simulink model "Ideal_Push_pull"  (R2022b)
settings: Solver=VariableStepAuto  StartTime=0.0  StopTime=0.1  FixedStep=1/2e6  RelTol=1e-3
libraries: spsSeriesRLCBranchLib x4, spsVoltageMeasurementLib x3, spsCurrentMeasurementLib x2, spsDiodeLib x2, spsIdealSwitchLib x2, spsDCVoltageSourceLib x1, spsGroundLib x1, spsMultiWindingTransformerLib x1, spspowerguiLib x1
settings Model: Creator=smlmc  LastModifiedBy=smlmc
settings DebuggingCC: MaskedZcDiagnostic=none  IgnoredZcDiagnostic=none

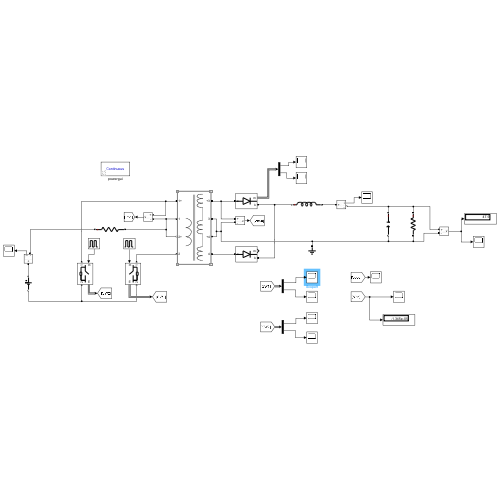
[thumbnail: Simulink's stored preview of the top-level diagram]
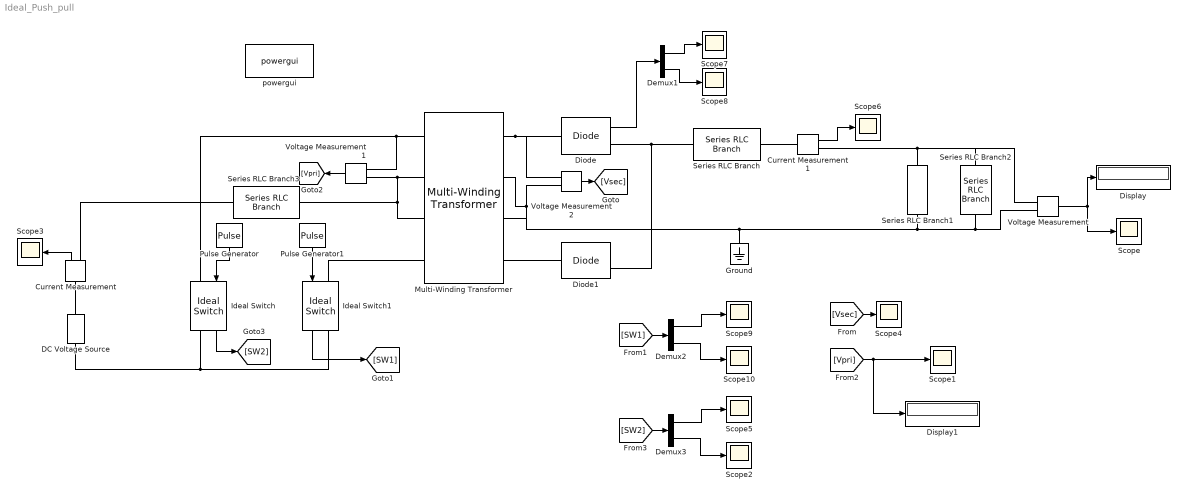
== system Ideal_Push_pull ==
  Current Measurement : spsCurrentMeasurementLib/Current Measurement  PhasorSimulation=off  OutputType=Complex  PSBequivalent=0
  Current Measurement1 : spsCurrentMeasurementLib/Current Measurement  PhasorSimulation=off  OutputType=Complex  PSBequivalent=0
  DC Voltage Source : spsDCVoltageSourceLib/DC Voltage Source  Amplitude=12  Measurements=None
  Demux1 : Demux  Outputs=2
  Demux2 : Demux  Outputs=2
  Demux3 : Demux  Outputs=2
  Diode : spsDiodeLib/Diode  Ron=0.001  Lon=0  Vf=0.1  IC=0  UseSnubber=0  Rs=inf  Cs=0  Measurements=on
  Diode1 : spsDiodeLib/Diode  Ron=0.001  Lon=0  Vf=0.1  IC=0  UseSnubber=0  Rs=inf  Cs=0  Measurements=on
  Display : Display
  Display1 : Display
  Ground : spsGroundLib/Ground  LConnTagsString=a
  Ideal Switch : spsIdealSwitchLib/Ideal Switch  Ron=0.0001  Lon=0  IC=0  Rs=1e5  Cs=inf  Measurements=on
  Ideal Switch1 : spsIdealSwitchLib/Ideal Switch  Ron=0.0001  Lon=0  IC=0  Rs=1e5  Cs=inf  Measurements=on
  Multi-Winding Transformer : spsMultiWindingTransformerLib/Multi-Winding Transformer  LeftWindings=2  RightWindings=2  TappedWindings=no taps  NumberOfTaps=2  SetSaturation=off  Hysteresis=off  DataFile='hysteresis.mat'  Measurements=None  UNITS=SI  NominalPower=[100 100e3]  NominalVoltages=[7 7 32 32]  WindingResistances=[5.8 5.8 54.9 54.9]*0.00  WindingInductances=[0 0 0 0]  Rm=7350  Lm=97.1e-6  Saturation=[0 0;60.609 1.5325e-15;25254 1.9412e-15]  SpecifyInitialFlux=off  InitialFlux=0  BreakLoop=off  DiscreteSolver=Trapezoidal iterative  DataType=on  TransfoNumber=1
  Pulse Generator : DiscretePulseGenerator  PulseType=Time based  Period=1/40e3  PulseWidth=43.75
  Pulse Generator1 : DiscretePulseGenerator  PulseType=Time based  Period=1/40e3  PulseWidth=43.75  PhaseDelay=1/80e3
  Scope{,1..10} (11 alike) : Scope
  Series RLC Branch : spsSeriesRLCBranchLib/Series RLC Branch  LConnTagsString=__new0  RConnTagsString=__new0  BranchType=L  Resistance=0.001  Inductance=4e-3  SetiL0=off  InitialCurrent=0  Capacitance=1e-6  Setx0=off  InitialVoltage=0  Measurements=Branch voltage and current
  Series RLC Branch1 : spsSeriesRLCBranchLib/Series RLC Branch  LConnTagsString=__new0  RConnTagsString=__new0  BranchType=C  Resistance=1  Inductance=1e-3  SetiL0=off  InitialCurrent=0  Capacitance=2e-8  Setx0=off  InitialVoltage=0  Measurements=None
  Series RLC Branch2 : spsSeriesRLCBranchLib/Series RLC Branch  LConnTagsString=__new0  RConnTagsString=__new0  BranchType=R  Resistance=48  Inductance=1e-3  SetiL0=off  InitialCurrent=0  Capacitance=1e-6  Setx0=off  InitialVoltage=0  Measurements=None
  Series RLC Branch3 : spsSeriesRLCBranchLib/Series RLC Branch  LConnTagsString=__new0  RConnTagsString=__new0  BranchType=R  Resistance=0.0001  Inductance=1e-3  SetiL0=off  InitialCurrent=0  Capacitance=1e-6  Setx0=off  InitialVoltage=0  Measurements=None
  Voltage Measurement : spsVoltageMeasurementLib/Voltage Measurement  PhasorSimulation=off  OutputType=Complex  PSBequivalent=0
  Voltage Measurement1 : spsVoltageMeasurementLib/Voltage Measurement  PhasorSimulation=off  OutputType=Complex  PSBequivalent=0
  Voltage Measurement2 : spsVoltageMeasurementLib/Voltage Measurement  PhasorSimulation=off  OutputType=Complex  PSBequivalent=0
  powergui : spspowerguiLib/powergui  Priority=1  SimulationMode=Continuous  SampleTime=50e-6  frequency=60  Iterations=50  frequencyindice=0  Pbase=100e6  ErrMax=1e-4  UnitsV=kV  UnitsW=MW  buscounter=0  FunctionMessages=off  echomessages=off  EnableUseOfTLC=off  CurrentSourceSwitches=off  DisableSnubberDevices=off  DisableRonSwitches=off  DisableVfSwitches=off  DisplayEquations=off  AutomaticDiscreteSolvers=off  SolverType=Tustin/Backward Euler (TBE)  Interpol=off  ExternalGateDelay=off  methode=off  Ts=100  x0status=blocks  SPID=on  SwTol=0  HookPort=off  NonlinearTolerance=1e-4  nMaxIteration=100  ContinueOnMaxIteration=off  RestoreLinks=warning  ResistiveCurrentMeasurement=off  Frange=[0:2:500]  Ylog=off  Xlog=on  ShowGrid=off  save=off  variable=ZData  structure=0  ZoomFFT=off  StartTime=0.0  cycles=1  DisplayStyle=1  fundamental=60  FreqAxis=off  MaxFrequency=1000  frequencyindicesteady=1  RmsSteady=1  display=off
  wires:
  Pulse Generator/1 -> Ideal Switch/1
  Demux1/2 -> Scope8/1
  Diode/1 -> Demux1/1
  Current Measurement/1 -> Scope3/1
  Voltage Measurement/1 -> Scope/1, Display/1
  Pulse Generator1/1 -> Ideal Switch1/1
  Current Measurement1/1 -> Scope6/1
  Demux1/1 -> Scope7/1
  Voltage Measurement2/1 -> [Vsec]
  [Vsec] -> Scope4/1
  Demux2/1 -> Scope9/1
  Demux2/2 -> Scope10/1
  [SW1] -> Demux2/1
  Ideal Switch1/1 -> [SW1]
  [Vpri] -> Scope1/1, Display1/1
  Voltage Measurement1/1 -> [Vpri]
  Ideal Switch/1 -> [SW2]
  [SW2] -> Demux3/1
  Demux3/2 -> Scope2/1
  Demux3/1 -> Scope5/1
  connections:
  Diode/RConn1 -- Diode1/RConn1 -- Series RLC Branch/LConn1
  Ideal Switch1/RConn1 -- Ideal Switch/RConn1 -- DC Voltage Source/LConn1
  Voltage Measurement/LConn2 -- Voltage Measurement2/LConn2 -- Multi-Winding Transformer/RConn2 -- Multi-Winding Transformer/RConn3 -- Ground/LConn1 -- Series RLC Branch1/RConn1 -- Series RLC Branch2/RConn1
  Series RLC Branch2/LConn1 -- Voltage Measurement/LConn1 -- Series RLC Branch1/LConn1 -- Current Measurement1/RConn1
  Voltage Measurement1/LConn1 -- Multi-Winding Transformer/LConn1 -- Ideal Switch/LConn1
  Multi-Winding Transformer/RConn1 -- Diode/LConn1 -- Voltage Measurement2/LConn1
  Current Measurement/RConn1 -- Series RLC Branch3/LConn1
  Multi-Winding Transformer/RConn4 -- Diode1/LConn1
  Current Measurement1/LConn1 -- Series RLC Branch/RConn1
  DC Voltage Source/RConn1 -- Current Measurement/LConn1
  Ideal Switch1/LConn1 -- Multi-Winding Transformer/LConn4
  Multi-Winding Transformer/LConn2 -- Series RLC Branch3/RConn1 -- Multi-Winding Transformer/LConn3 -- Voltage Measurement1/LConn2
